simulink model "ADCCalibrationCAN"  (R2026a)
settings: Solver=FixedStepAuto  StopTime=inf  FixedStep=Ts_CPU  EnableMultiTasking=on
InitFcn:
  | Ts = 1e-4;
  | Tcpu = 50e-6; %Controller sample time
  | 
  | % PMSM parameters
  | PM = 0.03; % Permanent magnet flux linkage
  | Ld = 2e-4;  % d-axis inductance
  | Lq = 2e-4;  % q-axis inductance
  | L0 = 2e-4;  % 0-axis inductance
  | Rs = 0.013; % Stator resistance
  | N = 6; % Number of pole pairs
  | J = 0.2; % Moment of inertia
  | 
  | % encoder parameters
  | numSlits = 2000; % number of slits
  | pulseSigOffset = 0; % index pulse signal offset
  | shaftInitPos = 0; % motor shaft initial position
  | 
  | % DAC parameters
  | gain = 0.1;
  | bias = 0;
  | 
  | % circuit parameters
  | Vdc = 48;
  | 
  | % real-time parameters
  | ts_FPGA_clk = 5e-9;
  | ts_FPGA_mdl = 1e-6;
  | 
  | % Real-time processor or embedded controller
  | RTorTTL = 1; % 1: Real-time processor,    0: embedded controller
  | 
  | % sample times
  | f_base = 200e6;
  | PWM_frequency = 20e3;
  | ts_FPGA_clk = 1/f_base;
  | ts_FPGA_mdl =1e-6;
undefined symbols (not defined in the file or in its folder): Foc_Ki_IxTcpu, Foc_Kp_I, IO334, IO334_iDAC_bias, IO334_iDAC_gain, Maxon_645604_J, Maxon_645604_lambda_pm, Maxon_645604_Ld, Maxon_645604_Lq, Maxon_645604_Np, Maxon_645604_Rs, Maxon_645604_StaticF, Maxon_645604_ViscousF, PMSM3P2LInverter_limited, PMSM_3P2L_Inverter_Plant, Ts_CAN_Tx, Ts_CPU, Ts_UI
libraries: speedgoatlib_hdlCoder_IO3xx x31, canmsglib x7, speedgoatlib_IO611 x3, pwm_cpulib x1, quadrature_cpulib x1, resolver_cpulib x1
(part 2 of 2)

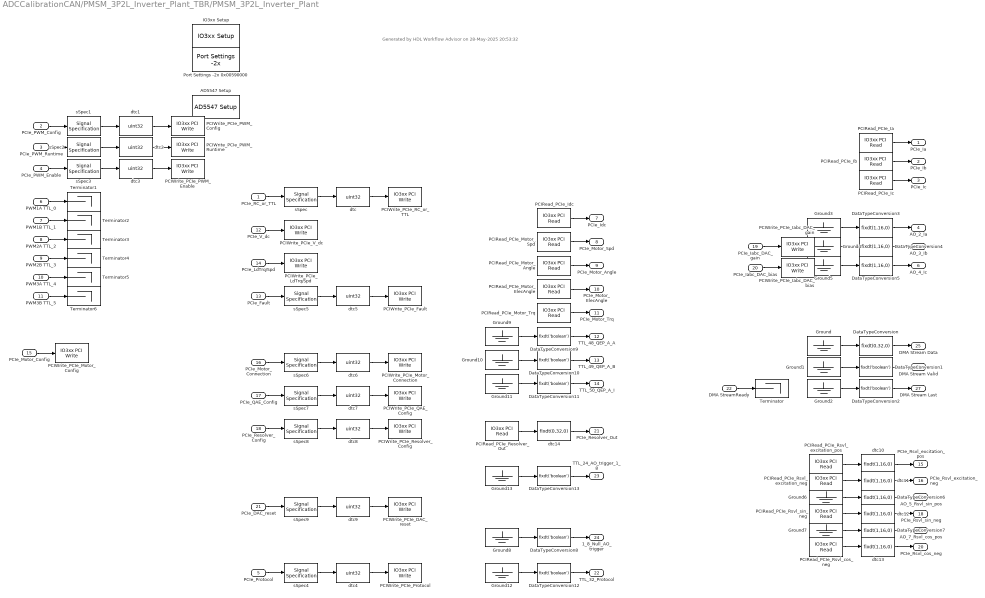
== system ADCCalibrationCAN/PMSM_3P2L_Inverter_Plant_TBR/PMSM_3P2L_Inverter_Plant ==
  note: Generated by HDL Workflow Advisor on 28-May-2025 20:53:32
  PCIe_RC_or_TTL : Inport
  PCIe_PWM_Config : Inport  Port=2
  PCIe_PWM_Runtime : Inport  Port=3
  PCIe_PWM_Enable : Inport  Port=4
  PCIe_Protocol : Inport  Port=5
  PWM1A TTL_0 : Inport  Port=6
  PWM1B TTL_1 : Inport  Port=7
  PWM2A TTL_2 : Inport  Port=8
  PWM2B TTL_3 : Inport  Port=9
  PWM3A TTL_4 : Inport  Port=10
  PWM3B TTL_5 : Inport  Port=11
  PCIe_V_dc : Inport  Port=12
  PCIe_Fault : Inport  Port=13
  PCIe_LdTrq/Spd : Inport  Port=14
  PCIe_Motor_Config : Inport  Port=15
  PCIe_Motor_Connection : Inport  Port=16
  PCIe_QAE_Config : Inport  Port=17
  PCIe_Resolver_Config : Inport  Port=18
  PCIe_Iabc_DAC_gain : Inport  Port=19
  PCIe_Iabc_DAC_bias : Inport  Port=20
  PCIe_DAC_reset : Inport  Port=21
  DMA StreamReady : Inport  Port=22
  AD5547 Setup : speedgoatlib_hdlCoder_IO3xx/AD5547 Setup  module_id=module_id  dacReset=on  dacGain_1=+/- 10.0V  dacActiv_1=off  dacInit_1=0  dacGain_2=+/- 2.5V  dacActiv_2=on  dacInit_2=0  dacGain_3=+/- 2.5V  dacActiv_3=on  dacInit_3=0  dacGain_4=+/- 2.5V  dacActiv_4=on  dacInit_4=0  dacGain_5=+/- 2.5V  dacActiv_5=on  dacInit_5=0  dacGain_6=+/- 10.0V  dacActiv_6=off  dacInit_6=0  dacGain_7=+/- 2.5V  dacActiv_7=on  dacInit_7=0  dacGain_8=+/- 10.0V  dacActiv_8=off  dacInit_8=0  dacGain_9=+/- 10.0V  dacActiv_9=off  dacInit_9=0  dacGain_10=+/- 10.0V  dacActiv_10=off  dacInit_10=0  dacGain_11=+/- 10.0V  dacActiv_11=off  dacInit_11=0  dacGain_12=+/- 10.0V  dacActiv_12=off  dacInit_12=0  dacGain_13=+/- 10.0V  dacActiv_13=off  dacInit_13=0  dacGain_14=+/- 10.0V  dacActiv_14=off  dacInit_14=0  dacGain_15=+/- 10.0V  dacActiv_15=off  dacInit_15=0  dacGain_16=+/- 10.0V  dacActiv_16=off  dacInit_16=0  dacGain_17=+/- 10.0V  dacActiv_17=off  dacInit_17=0  dacGain_18=+/- 10.0V  dacActiv_18=off  dacInit_18=0  dacGain_19=+/- 10.0V  dacActiv_19=off  dacInit_19=0  dacGain_20=+/- 10.0V  dacActiv_20=off  dacInit_20=0  dacGain_21=+/- 10.0V  dacActiv_21=off  dacInit_21=0  dacGain_22=+/- 10.0V  dacActiv_22=off  dacInit_22=0  dacGain_23=+/- 10.0V  dacActiv_23=off  dacInit_23=0  dacGain_24=+/- 10.0V  dacActiv_24=off  dacInit_24=0  dacGain_25=+/- 10.0V  dacActiv_25=off  dacInit_25=0  dacGain_26=+/- 10.0V  dacActiv_26=off  dacInit_26=0  dacGain_27=+/- 10.0V  dacActiv_27=off  dacInit_27=0  dacGain_28=+/- 10.0V  dacActiv_28=off  dacInit_28=0  dacGain_29=+/- 10.0V  dacActiv_29=off  dacInit_29=0  dacGain_30=+/- 10.0V  dacActiv_30=off  dacInit_30=0  dacGain_31=+/- 10.0V  dacActiv_31=off  dacInit_31=0  dacGain_32=+/- 10.0V  dacActiv_32=off  dacInit_32=0
  DataTypeConversion : DataTypeConversion  OutDataTypeStr=fixdt(0,32,0)  ConvertRealWorld=Stored Integer (SI)  SaturateOnIntegerOverflow=off  RndMeth=Floor
  DataTypeConversion{1..2,8..13} (8 alike) : DataTypeConversion  OutDataTypeStr=fixdt('boolean')  ConvertRealWorld=Stored Integer (SI)  SaturateOnIntegerOverflow=off  RndMeth=Floor
  DataTypeConversion{3..7} (5 alike) : DataTypeConversion  OutDataTypeStr=fixdt(1,16,0)  ConvertRealWorld=Stored Integer (SI)  SaturateOnIntegerOverflow=off  RndMeth=Floor
  Ground{,1..13} (14 alike) : Ground
  IO3xx Setup : speedgoatlib_hdlCoder_IO3xx/IO3xx Setup  mdl_ss_name=PMSM3P2LInverter_limited/PMSM_3P2L_Inverter_Plant  board_type=IO334-325k  fpga_sync_mode=on  reset_mode=on  reset_mode_stop=on  device_id=1  module_id=module_id  pci_slot=slot  fpga_mat_file=c:\hdl_prj\hdlsrc\PMSM3P2LInverter_limited\PMSM_3P2L_Inverter_Plant.mat  timestamp_mcs=05/28/25 20:27:22  timestamp=3803399894  tsreg=hex2dec('8')  bsf_file=PMSM_3P2L_Inverter_Plant_2505281921.mcs  mcs=0  init_reg_list=[]
  PCIRead_PCIe_Ia : speedgoatlib_hdlCoder_IO3xx/IO3xx PCI Read  device_id=1  module_id=module_id  board_type=IO334-325k  port_name=PCIe_Ia  port_offset=hex2dec('128')  port_type=single  port_dim=1  strobe=0  sample_time=ts
  PCIRead_PCIe_Ib : speedgoatlib_hdlCoder_IO3xx/IO3xx PCI Read  device_id=1  module_id=module_id  board_type=IO334-325k  port_name=PCIe_Ib  port_offset=hex2dec('12C')  port_type=single  port_dim=1  strobe=0  sample_time=ts
  PCIRead_PCIe_Ic : speedgoatlib_hdlCoder_IO3xx/IO3xx PCI Read  device_id=1  module_id=module_id  board_type=IO334-325k  port_name=PCIe_Ic  port_offset=hex2dec('130')  port_type=single  port_dim=1  strobe=0  sample_time=ts
  PCIRead_PCIe_Idc : speedgoatlib_hdlCoder_IO3xx/IO3xx PCI Read  device_id=1  module_id=module_id  board_type=IO334-325k  port_name=PCIe_Idc  port_offset=hex2dec('134')  port_type=single  port_dim=1  strobe=0  sample_time=ts
  PCIRead_PCIe_Motor_Angle : speedgoatlib_hdlCoder_IO3xx/IO3xx PCI Read  device_id=1  module_id=module_id  board_type=IO334-325k  port_name=PCIe_Motor_Angle  port_offset=hex2dec('13C')  port_type=single  port_dim=1  strobe=0  sample_time=ts
  PCIRead_PCIe_Motor_ElecAngle : speedgoatlib_hdlCoder_IO3xx/IO3xx PCI Read  device_id=1  module_id=module_id  board_type=IO334-325k  port_name=PCIe_Motor_ElecAngle  port_offset=hex2dec('184')  port_type=single  port_dim=1  strobe=0  sample_time=ts
  PCIRead_PCIe_Motor_Spd : speedgoatlib_hdlCoder_IO3xx/IO3xx PCI Read  device_id=1  module_id=module_id  board_type=IO334-325k  port_name=PCIe_Motor_Spd  port_offset=hex2dec('138')  port_type=single  port_dim=1  strobe=0  sample_time=ts
  PCIRead_PCIe_Motor_Trq : speedgoatlib_hdlCoder_IO3xx/IO3xx PCI Read  device_id=1  module_id=module_id  board_type=IO334-325k  port_name=PCIe_Motor_Trq  port_offset=hex2dec('188')  port_type=single  port_dim=1  strobe=0  sample_time=ts
  PCIRead_PCIe_Resolver_Out : speedgoatlib_hdlCoder_IO3xx/IO3xx PCI Read  device_id=1  module_id=module_id  board_type=IO334-325k  port_name=PCIe_Resolver_Out  port_offset=hex2dec('1D0')  port_type=uint32  port_dim=3  strobe=hex2dec('1E0')  sample_time=ts
  PCIRead_PCIe_Rsvl_cos_neg : speedgoatlib_hdlCoder_IO3xx/IO3xx PCI Read  device_id=1  module_id=module_id  board_type=IO334-325k  port_name=PCIe_Rsvl_cos_neg  port_offset=hex2dec('198')  port_type=uint32  port_dim=1  strobe=0  sample_time=ts
  PCIRead_PCIe_Rsvl_excitation_neg : speedgoatlib_hdlCoder_IO3xx/IO3xx PCI Read  device_id=1  module_id=module_id  board_type=IO334-325k  port_name=PCIe_Rsvl_excitation_neg  port_offset=hex2dec('190')  port_type=uint32  port_dim=1  strobe=0  sample_time=ts
  PCIRead_PCIe_Rsvl_excitation_pos : speedgoatlib_hdlCoder_IO3xx/IO3xx PCI Read  device_id=1  module_id=module_id  board_type=IO334-325k  port_name=PCIe_Rsvl_excitation_pos  port_offset=hex2dec('194')  port_type=uint32  port_dim=1  strobe=0  sample_time=ts
  PCIRead_PCIe_Rsvl_sin_neg : speedgoatlib_hdlCoder_IO3xx/IO3xx PCI Read  device_id=1  module_id=module_id  board_type=IO334-325k  port_name=PCIe_Rsvl_sin_neg  port_offset=hex2dec('18C')  port_type=uint32  port_dim=1  strobe=0  sample_time=ts
  PCIWrite_PCIe_DAC_reset : speedgoatlib_hdlCoder_IO3xx/IO3xx PCI Write  device_id=1  module_id=module_id  board_type=IO334-325k  port_name=PCIe_DAC_reset  port_offset=hex2dec('124')  port_type=uint32  port_dim=1  strobe=0  sample_time=ts
  PCIWrite_PCIe_Fault : speedgoatlib_hdlCoder_IO3xx/IO3xx PCI Write  device_id=1  module_id=module_id  board_type=IO334-325k  port_name=PCIe_Fault  port_offset=hex2dec('110')  port_type=uint32  port_dim=1  strobe=0  sample_time=ts
  PCIWrite_PCIe_Iabc_DAC_bias : speedgoatlib_hdlCoder_IO3xx/IO3xx PCI Write  device_id=1  module_id=module_id  board_type=IO334-325k  port_name=PCIe_Iabc_DAC_bias  port_offset=hex2dec('120')  port_type=single  port_dim=1  strobe=0  sample_time=ts
  PCIWrite_PCIe_Iabc_DAC_gain : speedgoatlib_hdlCoder_IO3xx/IO3xx PCI Write  device_id=1  module_id=module_id  board_type=IO334-325k  port_name=PCIe_Iabc_DAC_gain  port_offset=hex2dec('11C')  port_type=single  port_dim=1  strobe=0  sample_time=ts
  PCIWrite_PCIe_LdTrq/Spd : speedgoatlib_hdlCoder_IO3xx/IO3xx PCI Write  device_id=1  module_id=module_id  board_type=IO334-325k  port_name=PCIe_LdTrq//Spd  port_offset=hex2dec('114')  port_type=single  port_dim=1  strobe=0  sample_time=ts
  PCIWrite_PCIe_Motor_Config : speedgoatlib_hdlCoder_IO3xx/IO3xx PCI Write  device_id=1  module_id=module_id  board_type=IO334-325k  port_name=PCIe_Motor_Config  port_offset=hex2dec('340')  port_type=single  port_dim=9  strobe=hex2dec('380')  sample_time=ts
  PCIWrite_PCIe_Motor_Connection : speedgoatlib_hdlCoder_IO3xx/IO3xx PCI Write  device_id=1  module_id=module_id  board_type=IO334-325k  port_name=PCIe_Motor_Connection  port_offset=hex2dec('118')  port_type=uint32  port_dim=1  strobe=0  sample_time=ts
  PCIWrite_PCIe_PWM_Config : speedgoatlib_hdlCoder_IO3xx/IO3xx PCI Write  device_id=1  module_id=module_id  board_type=IO334-325k  port_name=PCIe_PWM_Config  port_offset=hex2dec('200')  port_type=uint32  port_dim=48  strobe=hex2dec('300')  sample_time=ts
  PCIWrite_PCIe_PWM_Enable : speedgoatlib_hdlCoder_IO3xx/IO3xx PCI Write  device_id=1  module_id=module_id  board_type=IO334-325k  port_name=PCIe_PWM_Enable  port_offset=hex2dec('104')  port_type=uint32  port_dim=1  strobe=0  sample_time=ts
  PCIWrite_PCIe_PWM_Runtime : speedgoatlib_hdlCoder_IO3xx/IO3xx PCI Write  device_id=1  module_id=module_id  board_type=IO334-325k  port_name=PCIe_PWM_Runtime  port_offset=hex2dec('140')  port_type=uint32  port_dim=15  strobe=hex2dec('180')  sample_time=ts
  PCIWrite_PCIe_Protocol : speedgoatlib_hdlCoder_IO3xx/IO3xx PCI Write  device_id=1  module_id=module_id  board_type=IO334-325k  port_name=PCIe_Protocol  port_offset=hex2dec('108')  port_type=uint32  port_dim=1  strobe=0  sample_time=ts
  PCIWrite_PCIe_QAE_Config : speedgoatlib_hdlCoder_IO3xx/IO3xx PCI Write  device_id=1  module_id=module_id  board_type=IO334-325k  port_name=PCIe_QAE_Config  port_offset=hex2dec('3C0')  port_type=uint32  port_dim=8  strobe=hex2dec('3E0')  sample_time=ts
  PCIWrite_PCIe_RC_or_TTL : speedgoatlib_hdlCoder_IO3xx/IO3xx PCI Write  device_id=1  module_id=module_id  board_type=IO334-325k  port_name=PCIe_RC_or_TTL  port_offset=hex2dec('100')  port_type=uint32  port_dim=1  strobe=0  sample_time=ts
  PCIWrite_PCIe_Resolver_Config : speedgoatlib_hdlCoder_IO3xx/IO3xx PCI Write  device_id=1  module_id=module_id  board_type=IO334-325k  port_name=PCIe_Resolver_Config  port_offset=hex2dec('480')  port_type=uint32  port_dim=17  strobe=hex2dec('500')  sample_time=ts
  PCIWrite_PCIe_V_dc : speedgoatlib_hdlCoder_IO3xx/IO3xx PCI Write  device_id=1  module_id=module_id  board_type=IO334-325k  port_name=PCIe_V_dc  port_offset=hex2dec('10C')  port_type=single  port_dim=1  strobe=0  sample_time=ts
  Port Settings -2x 0x00590000 : speedgoatlib_hdlCoder_IO3xx/Port Settings -2x  module_id=module_id  rearIO=-21  PullRPort0=pull-up 3.3V  VioPort0=3.3V  PullRPort1=pull-up 3.3V  VioPort1=3.3V  PullRPort2=pull-up 3.3V  VioPort2=3.3V  PullRPort3=pull-up 3.3V  VioPort3=3.3V  PullRPort4=pull-up 3.3V  VioPort4=3.3V  PullRPort5=pull-up 3.3V  VioPort5=3.3V  PullRPort6=pull-up 3.3V  VioPort6=3.3V  I2cAddrOffset=5832704  DutAddrOffset=120
  Terminator{,1..6} (7 alike) : Terminator
  dtc{,1..9} (10 alike) : DataTypeConversion  OutDataTypeStr=uint32  ConvertRealWorld=Stored Integer (SI)  SaturateOnIntegerOverflow=off
  dtc{10..13} (4 alike) : DataTypeConversion  OutDataTypeStr=fixdt(1,16,0)  ConvertRealWorld=Stored Integer (SI)  SaturateOnIntegerOverflow=off
  dtc14 : DataTypeConversion  OutDataTypeStr=fixdt(0,32,0)  ConvertRealWorld=Stored Integer (SI)  SaturateOnIntegerOverflow=off
  sSpec{,3..4,6} (4 alike) : SignalSpecification  OutDataTypeStr=fixdt('boolean')
  sSpec{1..2,5,7..8} (5 alike) : SignalSpecification  OutDataTypeStr=fixdt(0,32,0)
  sSpec9 : SignalSpecification  OutDataTypeStr=fixdt(0,16,0)
  PCIe_Ia : Outport
  PCIe_Ib : Outport  Port=2
  PCIe_Ic : Outport  Port=3
  AO_2_Ia : Outport  Port=4
  AO_3_Ib : Outport  Port=5
  AO_4_Ic : Outport  Port=6
  PCIe_Idc : Outport  Port=7
  PCIe_Motor_Spd : Outport  Port=8
  PCIe_Motor_Angle : Outport  Port=9
  PCIe_Motor_ElecAngle : Outport  Port=10
  PCIe_Motor_Trq : Outport  Port=11
  TTL_48_QEP_A_A : Outport  Port=12
  TTL_49_QEP_A_B : Outport  Port=13
  "TTL_50_QEP_A_I   " : Outport  Port=14
  PCIe_Rsvl_excitation_pos : Outport  Port=15
  PCIe_Rsvl_excitation_neg : Outport  Port=16
  AO_5_Rsvl_sin_pos : Outport  Port=17
  PCIe_Rsvl_sin_neg : Outport  Port=18
  AO_7_Rsvl_cos_pos : Outport  Port=19
  PCIe_Rsvl_cos_neg : Outport  Port=20
  PCIe_Resolver_Out : Outport  Port=21
  TTL_32_Protocol : Outport  Port=22
  TTL_24_AO_trigger_1_8 : Outport  Port=23
  1_8_Null_AO_trigger : Outport  Port=24
  DMA Stream Data : Outport  Port=25
  DMA Stream Valid : Outport  Port=26
  DMA Stream Last : Outport  Port=27
  wires:
  PCIe_RC_or_TTL/1 -> sSpec/1
  sSpec/1 -> dtc/1
  dtc/1 -> PCIWrite_PCIe_RC_or_TTL/1
  PCIe_PWM_Config/1 -> sSpec1/1
  sSpec1/1 -> dtc1/1
  dtc1/1 -> PCIWrite_PCIe_PWM_Config/1
  PCIe_PWM_Runtime/1 -> sSpec2/1
  sSpec2/1 -> dtc2/1
  dtc2/1 -> PCIWrite_PCIe_PWM_Runtime/1
  PCIe_PWM_Enable/1 -> sSpec3/1
  sSpec3/1 -> dtc3/1
  dtc3/1 -> PCIWrite_PCIe_PWM_Enable/1
  PCIe_Protocol/1 -> sSpec4/1
  sSpec4/1 -> dtc4/1
  dtc4/1 -> PCIWrite_PCIe_Protocol/1
  PCIe_V_dc/1 -> PCIWrite_PCIe_V_dc/1
  PCIe_Fault/1 -> sSpec5/1
  sSpec5/1 -> dtc5/1
  dtc5/1 -> PCIWrite_PCIe_Fault/1
  PCIe_LdTrq/Spd/1 -> PCIWrite_PCIe_LdTrq/Spd/1
  PCIe_Motor_Config/1 -> PCIWrite_PCIe_Motor_Config/1
  PCIe_Motor_Connection/1 -> sSpec6/1
  sSpec6/1 -> dtc6/1
  dtc6/1 -> PCIWrite_PCIe_Motor_Connection/1
  PCIe_QAE_Config/1 -> sSpec7/1
  sSpec7/1 -> dtc7/1
  dtc7/1 -> PCIWrite_PCIe_QAE_Config/1
  PCIe_Resolver_Config/1 -> sSpec8/1
  sSpec8/1 -> dtc8/1
  dtc8/1 -> PCIWrite_PCIe_Resolver_Config/1
  PCIe_Iabc_DAC_gain/1 -> PCIWrite_PCIe_Iabc_DAC_gain/1
  PCIe_Iabc_DAC_bias/1 -> PCIWrite_PCIe_Iabc_DAC_bias/1
  PCIe_DAC_reset/1 -> sSpec9/1
  sSpec9/1 -> dtc9/1
  dtc9/1 -> PCIWrite_PCIe_DAC_reset/1
  PCIRead_PCIe_Ia/1 -> PCIe_Ia/1
  PCIRead_PCIe_Ib/1 -> PCIe_Ib/1
  PCIRead_PCIe_Ic/1 -> PCIe_Ic/1
  PCIRead_PCIe_Idc/1 -> PCIe_Idc/1
  PCIRead_PCIe_Motor_Spd/1 -> PCIe_Motor_Spd/1
  PCIRead_PCIe_Motor_Angle/1 -> PCIe_Motor_Angle/1
  PCIRead_PCIe_Motor_ElecAngle/1 -> PCIe_Motor_ElecAngle/1
  PCIRead_PCIe_Motor_Trq/1 -> PCIe_Motor_Trq/1
  dtc10/1 -> PCIe_Rsvl_excitation_pos/1
  PCIRead_PCIe_Rsvl_excitation_pos/1 -> dtc10/1
  dtc11/1 -> PCIe_Rsvl_excitation_neg/1
  PCIRead_PCIe_Rsvl_excitation_neg/1 -> dtc11/1
  dtc12/1 -> PCIe_Rsvl_sin_neg/1
  PCIRead_PCIe_Rsvl_sin_neg/1 -> dtc12/1
  dtc13/1 -> PCIe_Rsvl_cos_neg/1
  PCIRead_PCIe_Rsvl_cos_neg/1 -> dtc13/1
  dtc14/1 -> PCIe_Resolver_Out/1
  PCIRead_PCIe_Resolver_Out/1 -> dtc14/1
  DMA StreamReady/1 -> Terminator/1
  DataTypeConversion/1 -> DMA Stream Data/1
  Ground/1 -> DataTypeConversion/1
  DataTypeConversion1/1 -> DMA Stream Valid/1
  Ground1/1 -> DataTypeConversion1/1
  DataTypeConversion2/1 -> DMA Stream Last/1
  Ground2/1 -> DataTypeConversion2/1
  DataTypeConversion3/1 -> AO_2_Ia/1
  Ground3/1 -> DataTypeConversion3/1
  DataTypeConversion4/1 -> AO_3_Ib/1
  Ground4/1 -> DataTypeConversion4/1
  DataTypeConversion5/1 -> AO_4_Ic/1
  Ground5/1 -> DataTypeConversion5/1
  DataTypeConversion6/1 -> AO_5_Rsvl_sin_pos/1
  Ground6/1 -> DataTypeConversion6/1
  DataTypeConversion7/1 -> AO_7_Rsvl_cos_pos/1
  Ground7/1 -> DataTypeConversion7/1
  DataTypeConversion8/1 -> 1_8_Null_AO_trigger/1
  Ground8/1 -> DataTypeConversion8/1
  PWM1A TTL_0/1 -> Terminator1/1
  PWM1B TTL_1/1 -> Terminator2/1
  PWM2A TTL_2/1 -> Terminator3/1
  PWM2B TTL_3/1 -> Terminator4/1
  PWM3A TTL_4/1 -> Terminator5/1
  PWM3B TTL_5/1 -> Terminator6/1
  DataTypeConversion9/1 -> TTL_48_QEP_A_A/1
  Ground9/1 -> DataTypeConversion9/1
  DataTypeConversion10/1 -> TTL_49_QEP_A_B/1
  Ground10/1 -> DataTypeConversion10/1
  DataTypeConversion11/1 -> "TTL_50_QEP_A_I   "/1
  Ground11/1 -> DataTypeConversion11/1
  DataTypeConversion12/1 -> TTL_32_Protocol/1
  Ground12/1 -> DataTypeConversion12/1
  DataTypeConversion13/1 -> TTL_24_AO_trigger_1_8/1
  Ground13/1 -> DataTypeConversion13/1
